simulink model "probthree"  (R2020b)
settings: Solver=VariableStepAuto  StartTime=0.0  StopTime=50  RelTol=1e-3
model workspace (MAT data in the model file):
  Kd = 346
  Ki = 76
  Kp = 1000
  N = 100000
  b = 50
  m = 1000
  u = 500
settings Model: DataDictionary=data.sldd  Creator=znome  LastModifiedBy='Z'ome
settings SimscapeCC: SimscapeNormalizeSystem=off

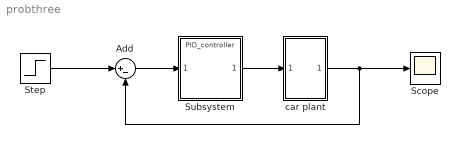
== system probthree ==
  Add : Sum  Inputs=|+-
  Scope : Scope
  Step : Step  Time=0  After=u  SampleTime=0
  Subsystem : ModelReference  ModelNameDialog=PID_controller  SimulationMode=Normal  ModelReferenceVersion=1.8
  car plant : Subsystem
  wires:
  Step/1 -> Add/1
  car plant/1(Out1) -> Scope/1, Add/2
  Add/1 -> Subsystem/1
  Subsystem/1 -> car plant/1(In1)

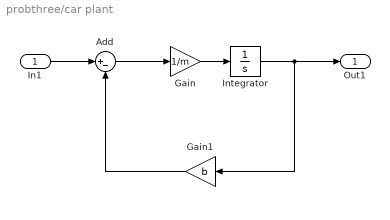
== system probthree/car plant ==
  In1 : Inport
  Add : Sum  Inputs=|+-
  Gain : Gain  Gain=1/m
  Gain1 : Gain  Gain=b
  Integrator : Integrator
  Out1 : Outport
  wires:
  Gain/1 -> Integrator/1
  Integrator/1 -> Out1/1, Gain1/1
  Gain1/1 -> Add/2
  In1/1 -> Add/1
  Add/1 -> Gain/1
